simulink model "FastBlockLMS"  (R2023b)
settings: Solver=ode3  StartTime=0.0  StopTime=inf  RelTol=1e-3  EnableMultiTasking=on
libraries: dspadpt3 x1, matrix_library x1, dspsrcs4 x1
settings Model: FPTRunName=Active  ExtModeTrigDuration=2  Creator=aaron  LastModifiedBy=aaron
settings SolverCC: AlgebraicLoopSolver=TrustRegion  PositivePriorityOrder=on
settings DataIOCC: LimitDataPoints=on  SaveFormat=Array
settings OptimizationCC: ExpressionDepthLimit=2147483647  LifeSpan=Inf  MaxStackSize=64
settings DebuggingCC: UnderspecifiedInitializationDetection=Classic  MergeDetectMultiDrivingBlocksExec=none  FcnCallInpInsideContextMsg=warning  UnconnectedInputMsg=warning  UnconnectedOutputMsg=warning  UnconnectedLineMsg=warning  AllowSymbolicDim=off  StateNameClashWarn=warning  SubsystemReferenceDiagnosticForUnitTest=warning  SFUnexpectedBacktrackingDiag=warning  SFNoUnconditionalDefaultTransitionDiag=warning  SFExecutionAtInitializationDiag=none  ArithmeticOperatorsInVariantConditions=warning
settings HardwareCC: ProdBitPerPointer=32  ProdBitPerSizeT=32  ProdBitPerPtrDiffT=32  ProdLargestAtomicInteger=Long  ProdLargestAtomicFloat=Double  ProdWordSize=32  ProdHWDeviceType=ARM Compatible->ARM Cortex  UseEmbeddedCoderFeatures=off  UseSimulinkCoderFeatures=off
settings ModelReferenceCC: EnableRefExpFcnMdlSchedulingChecks=on  PropagateSignalLabelsOutOfModel=off
settings SFSimCC: SimUseLocalCustomCode=off  CustomCodeUndefinedFunction=UseInterfaceOnly
settings RTWCC: Description=Embedded Coder  SystemTargetFile=ert.tlc  HardwareBoard=Raspberry Pi  TemplateMakefile=ert_default_tmf  GenerateReport=on  RTWVerbose=off  RTWUseLocalCustomCode=off  Toolchain=GNU GCC Embedded Linux  BuildConfiguration=Faster Runs  LaunchReport=on
settings CodeAppCC: ForceParamTrailComments=on  OperatorAnnotations=on  StateflowObjectComments=on  MATLABSourceComments=on
settings ERTTargetCC: MultiwordLength=2048  ERTCustomFileBanners=off  SupportContinuousTime=on  SupportNonInlinedSFcns=on  RemoveResetFunc=off  SupportVariableSizeSignals=on  ModelStepFunctionPrototypeControlCompliant=off
settings ConfigComp: CovMetricSettings=dw  CovSaveCumulativeToWorkspaceVar=on  CovSaveSingleToWorkspaceVar=on  CovExternalEMLEnable=off  CovSFcnEnable=off

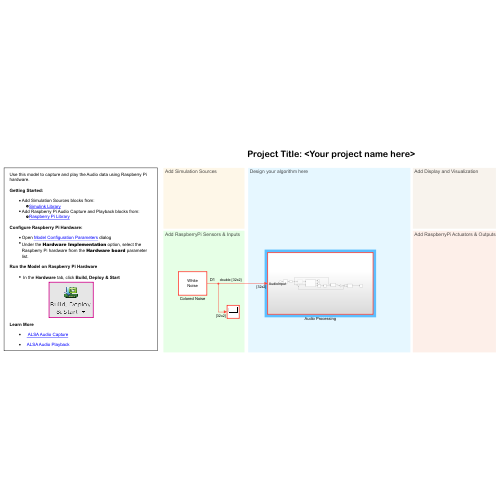
[thumbnail: Simulink's stored preview of the top-level diagram]
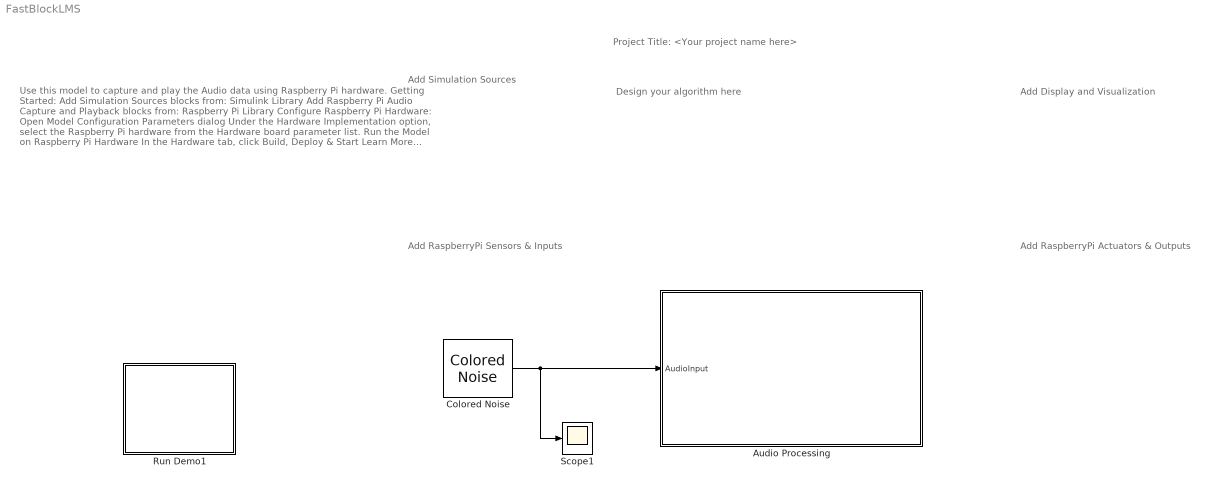
== system FastBlockLMS ==
  note: Use this model to capture and play the Audio data using Raspberry Pi hardware.
      |
      | Getting Started:
      |
      | Add Simulation Sources blocks from:
      | Simulink Library
      | Add Raspberry Pi Audio Capture and Playback blocks from:
      | Raspberry Pi Library
      |
      | Configure Raspberry Pi Hardware:
      |
      | Open Model Configuration Parameters dialog
      | Under the Hardware Implementation option, select the Raspberry Pi hardware from the Hardware board parameter list.
      |
      | Run the Model on Raspberry Pi Hardware
      |
      | In the Hardware tab, click Build, Deploy & Start
      |
      | Learn More
      | ALSA Audio Capture
      | ALSA Audio Playback
  note: Add Simulation Sources
  note: Add Display and Visualization
  note: Design your algorithm here
  note: Add RaspberryPi Actuators & Outputs
  note: Project Title: <Your project name here>
  note: Add RaspberryPi Sensors & Inputs
  Audio Processing : Subsystem
  Colored Noise : dspsrcs4/Colored Noise  Color=white  InverseFrequencyPower=1  BoundedOutput=off  NumChannels=2  OutputDataType=double  SamplesPerFrame=32  SampleTime=1/44100  RandomStream=mt19937ar with seed  Seed=67  SimulateUsing=Interpreted execution
      settings: LibrarySourceBlock=audiosources/Colored Noise
  Run Demo1 : Subsystem  Description=Controls host-side RTDX processing.
      mask Display: pic=imread('raspberrypiBuildDeployAndStart.png');image(pic);
  Scope1 : Scope
  wires:
  Colored Noise/1 -> Scope1/1, Audio Processing/1(AudioInput)

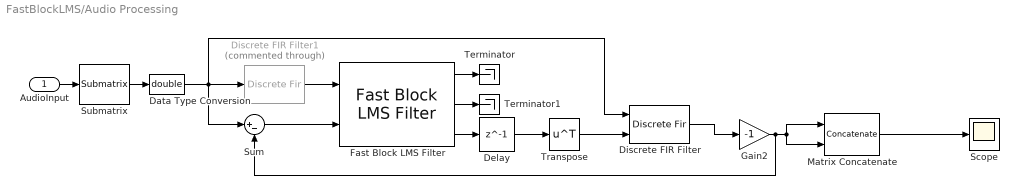
== system FastBlockLMS/Audio Processing ==
  AudioInput : Inport
  Data Type Conversion : DataTypeConversion  OutDataTypeStr=double  SaturateOnIntegerOverflow=off  RndMeth=Floor
  Delay : Delay  DelayLength=1  InitialCondition=0
  Discrete FIR Filter : DiscreteFir  CoefSource=Input port
      settings: InputPortMap=u0,u1
  Discrete FIR Filter1 : DiscreteFir  Commented=through  Coefficients="[0.466  0.533  -0.257  -0.274  -0.231  -0.175]"
  Fast Block LMS Filter : dspadpt3/Fast Block LMS Filter  algo=Fast Block LMS  L=32  N=32  stepflag=Dialog  mu=0.008  leakage=1.0  addnparflag=on  ic=0  Adapt=off  resetflag=None  weights=on
  Gain2 : Gain  Gain=-1  OutDataTypeStr=double
  Matrix Concatenate : Concatenate  Mode=Multidimensional array  ConcatenateDimension=2
  Scope : Scope
  Submatrix : matrix_library/Submatrix  RowSpan=Range of rows  RowStartMode=First  RowStartIndex=1  RowEndMode=Last  RowEndIndex=1  ColSpan=One column  ColStartMode=First  ColStartIndex=1  ColEndMode=Last  ColEndIndex=1
  Sum : Sum  Inputs=|+-
  Terminator : Terminator
  Terminator1 : Terminator
  Transpose : Math  Operator=transpose
  wires:
  AudioInput/1 -> Submatrix/1
  Submatrix/1 -> Data Type Conversion/1
  Matrix Concatenate/1 -> Scope/1
  Fast Block LMS Filter/3 -> Delay/1
  Delay/1 -> Transpose/1
  Discrete FIR Filter/1 -> Gain2/1
  Fast Block LMS Filter/2 -> Terminator1/1
  Fast Block LMS Filter/1 -> Terminator/1
  Transpose/1 -> Discrete FIR Filter/2
  Discrete FIR Filter1/1 -> Fast Block LMS Filter/1
  Data Type Conversion/1 -> Sum/1, Discrete FIR Filter/1, Discrete FIR Filter1/1
  Gain2/1 -> Sum/2, Matrix Concatenate/1, Matrix Concatenate/2
  Sum/1 -> Fast Block LMS Filter/2

== system FastBlockLMS/Run Demo1 ==
